simulink library "ReceiveFromBMS"  (R2016b)
settings: Solver=VariableStepAuto  StartTime=0.0  StopTime=10.0  RelTol=1e-3
settings Model: Creator=Nathan  LastModifiedBy=march

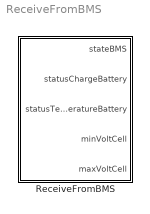
== system ReceiveFromBMS ==
  ReceiveFromBMS : Subsystem

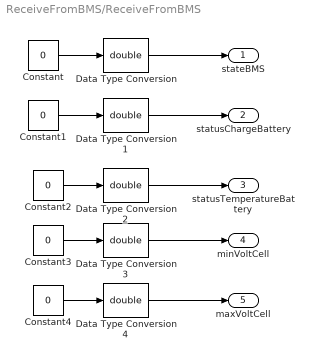
== system ReceiveFromBMS/ReceiveFromBMS ==
  Constant{,1..4} (5 alike) : Constant  Value=0
  Data Type Conversion{,1..4} (5 alike) : DataTypeConversion  OutDataTypeStr=double
  stateBMS : Outport
  statusChargeBattery : Outport  Port=2
  statusTemperatureBattery : Outport  Port=3
  minVoltCell : Outport  Port=4
  maxVoltCell : Outport  Port=5
  wires:
  Constant4/1 -> Data Type Conversion4/1
  Constant3/1 -> Data Type Conversion3/1
  Constant2/1 -> Data Type Conversion2/1
  Constant1/1 -> Data Type Conversion1/1
  Constant/1 -> Data Type Conversion/1
  Data Type Conversion/1 -> stateBMS/1
  Data Type Conversion1/1 -> statusChargeBattery/1
  Data Type Conversion2/1 -> statusTemperatureBattery/1
  Data Type Conversion3/1 -> minVoltCell/1
  Data Type Conversion4/1 -> maxVoltCell/1
